simulink model "Copy_of_Carrier_Phase_Shift"  (R2021a)
settings: Solver=FixedStepAuto  StartTime=0.0  StopTime=0.01  FixedStep=1e-7  MaxStep=1e-7  RelTol=1e-6
InitFcn:
  | fsw=50e3;
  | ma=0.5;
  | ffund=100;
  | 
  | L1=63e-6;
  | L2=50e-6;
  | M=18e-6;
  | C1=12.2e-9;
  | C2=14.5e-9;
  | R=20;
  | 
  | sn3=C1*C2*M*R;
  | sd4=C1*C2*L1*L2+C1*C2*L1*M+C1*C2*L2*M;
  | sd3= C1*C2*L1*R+ C1*C2*M*R;
  | sd2= C1*L1+C2*L2+C1*M+C2*M;
  | sd1=C2*R;
  | sd0=1;
libraries: spsSeriesRLCBranchLib x9, spsDiodeLib x4, spsVoltageMeasurementLib x3, spsControlledVoltageSourceLib x1, spsCurrentMeasurementLib x1, dspsigops x1, spspowerguiLib x1
settings Model: Creator=enes_  LastModifiedBy=enes_
settings DataIOCC: SaveFormat=StructureWithTime  ReturnWorkspaceOutputs=off

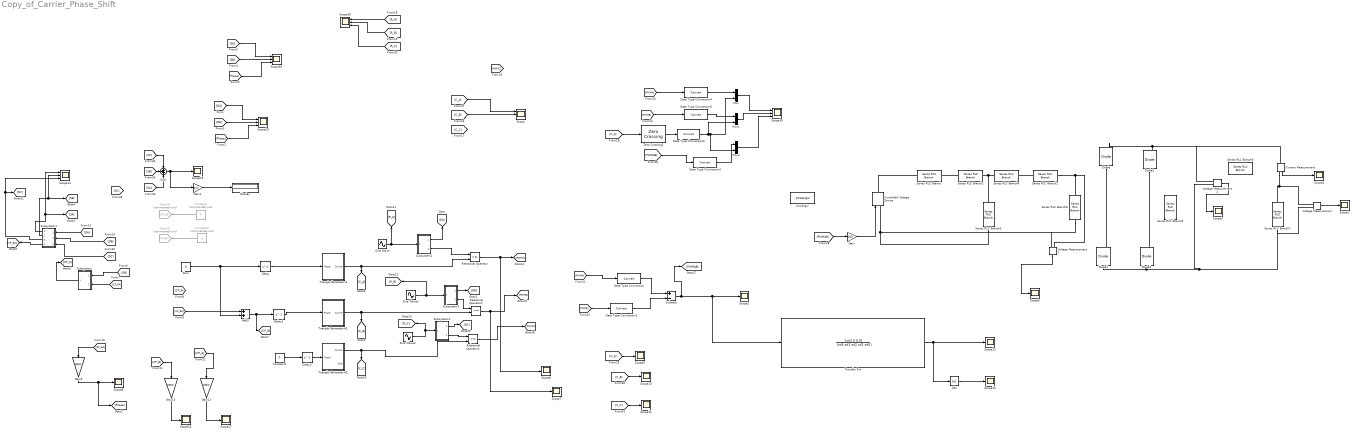
== system Copy_of_Carrier_Phase_Shift ==
  Abs : Abs
  Add3 : Sum
  Constant : Constant  Commented=on  Value=0
  Constant1 : Constant  Value=0
  Constant2 : Constant  Commented=on  Value=pi
  Controlled Voltage Source : spsControlledVoltageSourceLib/Controlled Voltage Source  Initialize=on  Source_Type=AC  Amplitude=0  Phase=0  Frequency=0  Measurements=None
  Current Measurement : spsCurrentMeasurementLib/Current Measurement  PhasorSimulation=off  OutputType=Complex  PSBequivalent=0
  Data Type Conversion{,1..2,4..6} (6 alike) : DataTypeConversion
  Delay : Delay  DelayLength=1
  Delay1 : Delay  DelayLength=1
  Delay2 : Delay  DelayLength=1
  Diode{,1..3} (4 alike) : spsDiodeLib/Diode  Ron=0.001  Lon=0  Vf=0.8  IC=0  UseSnubber=0  Rs=500  Cs=250e-9  Measurements=on
  Display : Display
  Gain : Gain  Gain=100
  Gain1 : Gain  Gain=pi/2
  Gain12 : Gain  Gain=180/pi
  Gain13 : Gain  Gain=180/pi
  Gain9 : Gain  Gain=180/pi
  Goto18 : Goto  Commented=on  GotoTag=CP_A
  Goto19 : Goto  Commented=on  GotoTag=CP_BA
  Mux : Mux  Inputs=2
  Mux1 : Mux  Inputs=2
  Mux2 : Mux  Inputs=2
  Relational Operator : RelationalOperator  OutDataTypeStr=boolean  RndMeth=Simplest
  Relational Operator1 : RelationalOperator  OutDataTypeStr=boolean  RndMeth=Simplest
  Relational Operator2 : RelationalOperator  OutDataTypeStr=boolean  RndMeth=Simplest
  Scope{,14,29..30,38..39} (6 alike) : Scope  NumInputPorts=3
  Scope{1..13,15..17} (16 alike) : Scope
  Series RLC Branch : spsSeriesRLCBranchLib/Series RLC Branch  LConnTagsString=__new0  RConnTagsString=__new0  BranchType=C  Resistance=1  Inductance=1e-3  SetiL0=off  InitialCurrent=0  Capacitance=12.2e-9  Setx0=off  InitialVoltage=0  Measurements=None
  Series RLC Branch1 : spsSeriesRLCBranchLib/Series RLC Branch  LConnTagsString=__new0  RConnTagsString=__new0  BranchType=C  Resistance=1  Inductance=1e-3  SetiL0=off  InitialCurrent=0  Capacitance=14.5e-9  Setx0=off  InitialVoltage=0  Measurements=None
  Series RLC Branch2 : spsSeriesRLCBranchLib/Series RLC Branch  LConnTagsString=__new0  RConnTagsString=__new0  BranchType=L  Resistance=1  Inductance=63e-6  SetiL0=off  InitialCurrent=0  Capacitance=1e-6  Setx0=off  InitialVoltage=0  Measurements=None
  Series RLC Branch3 : spsSeriesRLCBranchLib/Series RLC Branch  LConnTagsString=__new0  RConnTagsString=__new0  BranchType=L  Resistance=1  Inductance=18e-6  SetiL0=off  InitialCurrent=0  Capacitance=1e-6  Setx0=off  InitialVoltage=0  Measurements=None
  Series RLC Branch4 : spsSeriesRLCBranchLib/Series RLC Branch  LConnTagsString=__new0  RConnTagsString=__new0  BranchType=L  Resistance=1  Inductance=50e-6  SetiL0=off  InitialCurrent=0  Capacitance=1e-6  Setx0=off  InitialVoltage=0  Measurements=None
  Series RLC Branch5 : spsSeriesRLCBranchLib/Series RLC Branch  LConnTagsString=__new0  RConnTagsString=__new0  BranchType=C  Resistance=1  Inductance=1e-3  SetiL0=off  InitialCurrent=0  Capacitance=100e-6  Setx0=off  InitialVoltage=0  Measurements=None
  Series RLC Branch6 : spsSeriesRLCBranchLib/Series RLC Branch  LConnTagsString=__new0  RConnTagsString=__new0  BranchType=L  Resistance=1  Inductance=500e-6  SetiL0=off  InitialCurrent=0  Capacitance=14.5e-9  Setx0=off  InitialVoltage=0  Measurements=None
  Series RLC Branch7 : spsSeriesRLCBranchLib/Series RLC Branch  LConnTagsString=__new0  RConnTagsString=__new0  BranchType=R  Resistance=40  Inductance=5e-3  SetiL0=off  InitialCurrent=0  Capacitance=1e-6  Setx0=off  InitialVoltage=0  Measurements=None
  Series RLC Branch8 : spsSeriesRLCBranchLib/Series RLC Branch  LConnTagsString=__new0  RConnTagsString=__new0  BranchType=R  Resistance=40  Inductance=5e-3  SetiL0=off  InitialCurrent=0  Capacitance=1e-6  Setx0=off  InitialVoltage=0  Measurements=None
  Sine Wave : Sin  Amplitude=ma  Frequency=2*pi*ffund  SampleTime=0
  Sine Wave1 : Sin  Amplitude=ma  Frequency=2*pi*ffund  Phase=2*pi/3  SampleTime=0
  Sine Wave2 : Sin  Amplitude=ma  Frequency=2*pi*ffund  Phase=-2*pi/3  SampleTime=0
  Subsystem : Subsystem
  Subsystem1 : Subsystem
  Subsystem2 : Subsystem
  Subsystem3 : Subsystem
  Subsystem4 : Subsystem
  Subtract : Sum  Inputs=+-
  Sum : Sum  Inputs=+++
  Transfer Fcn : TransferFcn  Numerator=[sn3 0 0 0]  Denominator=[sd4 sd3 sd2 sd1 sd0]
  Triangle Generator-A : Subsystem
  Triangle Generator-A1 : Subsystem
  Triangle Generator-A2 : Subsystem
  Voltage Measurement : spsVoltageMeasurementLib/Voltage Measurement  PhasorSimulation=off  OutputType=Complex  PSBequivalent=0
  Voltage Measurement1 : spsVoltageMeasurementLib/Voltage Measurement  PhasorSimulation=off  OutputType=Complex  PSBequivalent=0
  Voltage Measurement2 : spsVoltageMeasurementLib/Voltage Measurement  PhasorSimulation=off  OutputType=Complex  PSBequivalent=0
  Zero : Constant  Value=0  OutDataTypeStr=Inherit: Inherit via back propagation
  Zero Crossing2 : dspsigops/Zero Crossing  InputProcessing=Columns as channels (frame based)
      settings: SourceProductBaseCode=DS
  powergui : spspowerguiLib/powergui  Priority=1  SimulationMode=Continuous  SampleTime=50e-6  frequency=60  Iterations=50  frequencyindice=0  Pbase=100e6  ErrMax=1e-4  UnitsV=kV  UnitsW=MW  buscounter=0  FunctionMessages=off  echomessages=off  EnableUseOfTLC=off  CurrentSourceSwitches=off  DisableSnubberDevices=off  DisableRonSwitches=off  DisableVfSwitches=off  DisplayEquations=off  AutomaticDiscreteSolvers=off  SolverType=Tustin/Backward Euler (TBE)  Interpol=off  ExternalGateDelay=off  methode=off  Ts=100  x0status=blocks  SPID=on  SwTol=0  HookPort=off  NonlinearTolerance=1e-4  nMaxIteration=100  ContinueOnMaxIteration=off  RestoreLinks=warning  ResistiveCurrentMeasurement=off  Frange=[0:2:500]  Ylog=off  Xlog=on  ShowGrid=off  save=off  variable=ZData  structure=0  ZoomFFT=off  StartTime=0.0  cycles=1  DisplayStyle=1  fundamental=60  FreqAxis=off  MaxFrequency=1000  frequencyindicesteady=1  RmsSteady=1  display=off
  wires:
  Triangle Generator-A2/1(Carrier) -> [C_C], Relational Operator2/2
  Relational Operator1/1 -> Scope7/1, [PWMB]
  Data Type Conversion/1 -> Subtract/1
  Data Type Conversion1/1 -> Subtract/2
  Constant1/1 -> Delay2/1
  Delay1/1 -> Triangle Generator-A1/1(Phase)
  Delay2/1 -> Triangle Generator-A2/1(Phase)
  Add3/1 -> [CP_B], Delay1/1
  Subtract/1 -> [PWMAB], Transfer Fcn/1, Scope2/1
  Delay/1 -> Triangle Generator-A/1(Phase)
  Gain9/1 -> [Phase], Scope8/1
  Gain12/1 -> Scope17/1
  Gain13/1 -> Scope16/1
  Sine Wave2/1 -> [R_C], Subsystem4/1(In1)
  [DA] -> Scope29/1
  [DB] -> Scope29/2
  [Phase] -> Scope29/3
  [SB] -> Scope30/2
  [Phase] -> Scope30/3
  [SA] -> Scope30/1
  Triangle Generator-A/1(Carrier) -> Relational Operator/2, [C_A]
  Zero Crossing2/1 -> Data Type Conversion6/1
  Subsystem/1(Out1) -> [CP_A]
  [SB] -> Subsystem/1(In1)
  [CP_BA] -> Subsystem/2(In2)
  [CP_BA] -> Add3/1
  [CP_BA] -> Gain9/1
  [CP_B] -> Gain13/1
  [CP_A] -> Gain12/1
  [DA] -> Subsystem1/1(In1)
  [DB] -> Subsystem1/2(In2)
  Subsystem1/1(Out1) -> Scope14/1, [SA]
  Subsystem1/4(Out3) -> [CP_BA]
  Subsystem2/1(Out1) -> [DA]
  Subsystem2/2(Out2) -> Relational Operator/1
  Triangle Generator-A1/1(Carrier) -> Relational Operator1/2, [C_B]
  Sine Wave1/1 -> [R_B], Subsystem3/1(In1)
  Subsystem3/1(Out1) -> [DB]
  Subsystem3/2(Out2) -> Relational Operator1/1
  Sine Wave/1 -> Subsystem2/1(In1), [R_A]
  [PWMA] -> Data Type Conversion4/1
  Mux/1 -> Scope39/1
  Mux1/1 -> Scope39/2
  Data Type Conversion4/1 -> Mux/1
  [PWMB] -> Data Type Conversion5/1
  Data Type Conversion5/1 -> Mux1/1
  Data Type Conversion6/1 -> Mux1/2, Mux2/2, Mux/2
  Relational Operator/1 -> Scope6/1, [PWMA]
  Relational Operator2/1 -> [PWMC]
  [PWMA] -> Data Type Conversion/1
  [PWMB] -> Data Type Conversion1/1
  [PWMAB] -> Data Type Conversion2/1
  Mux2/1 -> Scope39/3
  Data Type Conversion2/1 -> Mux2/1
  [C_A] -> Zero Crossing2/1
  [C_A] -> Scope/1
  [C_B] -> Scope/2
  [PWMAB] -> Gain/1
  Gain/1 -> Controlled Voltage Source/1
  Voltage Measurement/1 -> Scope1/1
  Voltage Measurement1/1 -> Scope3/1
  Current Measurement/1 -> Scope4/1
  Voltage Measurement2/1 -> Scope5/1
  [R_B] -> Scope38/2
  [R_C] -> Scope38/3
  [R_A] -> Scope38/1
  Constant/1 -> Goto18/1
  Constant2/1 -> Goto19/1
  [C_A] -> Scope9/1
  [C_B] -> Scope10/1
  [C_C] -> Scope11/1
  Transfer Fcn/1 -> Abs/1, Scope12/1
  Abs/1 -> Scope13/1
  Zero/1 -> Add3/2, Delay/1
  Subsystem1/2(Out2) -> Scope14/2, [SB]
  Subsystem4/2(Out2) -> Relational Operator2/1
  Subsystem4/1(Out1) -> [DC]
  [DC] -> Subsystem1/3(In3)
  Subsystem1/3(Out4) -> Scope14/3, [SC]
  [SA] -> Sum/3
  [SB] -> Sum/2
  [SC] -> Sum/1
  Sum/1 -> Gain1/1, Scope15/1
  Gain1/1 -> Display/1
  connections:
  Series RLC Branch/LConn1 -- Controlled Voltage Source/RConn1
  Series RLC Branch2/LConn1 -- Series RLC Branch/RConn1
  Series RLC Branch3/LConn1 -- Series RLC Branch4/LConn1 -- Series RLC Branch2/RConn1
  Series RLC Branch1/LConn1 -- Series RLC Branch4/RConn1
  Series RLC Branch1/RConn1 -- Series RLC Branch8/LConn1 -- Voltage Measurement2/LConn1
  Series RLC Branch3/RConn1 -- Series RLC Branch8/RConn1 -- Voltage Measurement2/LConn2 -- Controlled Voltage Source/LConn1
  Diode/RConn1 -- Current Measurement/LConn1 -- Voltage Measurement1/LConn1 -- Diode2/RConn1
  Diode1/LConn1 -- Voltage Measurement1/LConn2 -- Voltage Measurement/LConn2 -- Series RLC Branch7/RConn1 -- Diode3/LConn1
  Voltage Measurement/LConn1 -- Current Measurement/RConn1 -- Series RLC Branch7/LConn1
  Diode/LConn1 -- Diode1/RConn1
  Diode2/LConn1 -- Diode3/RConn1

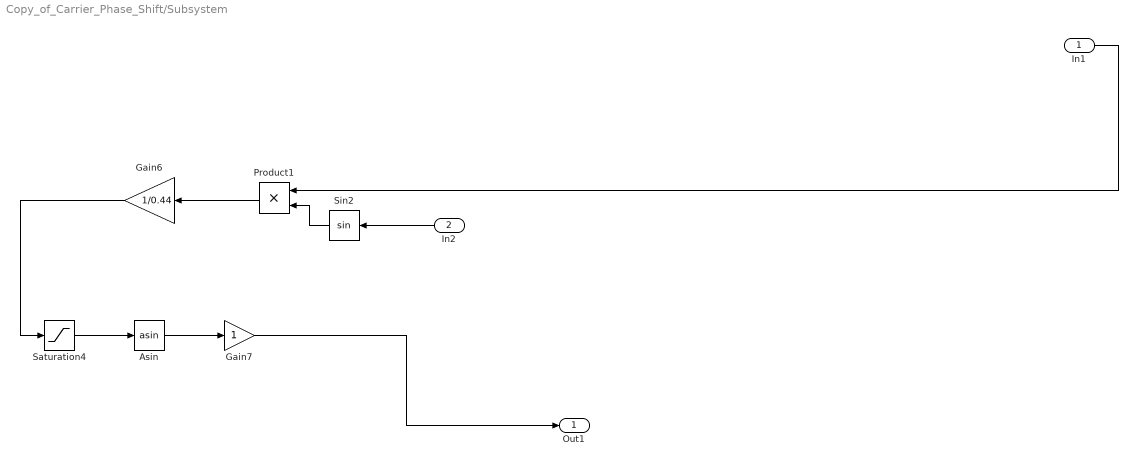
== system Copy_of_Carrier_Phase_Shift/Subsystem ==
  In1 : Inport
  In2 : Inport  Port=2
  Asin : Trigonometry  Operator=asin
  Gain6 : Gain  Gain=1/0.44
  Gain7 : Gain
  Product1 : Product
  Saturation4 : Saturate  UpperLimit=1  LowerLimit=-1
  Sin2 : Trigonometry
  Out1 : Outport
  wires:
  In2/1 -> Sin2/1
  Saturation4/1 -> Asin/1
  Gain7/1 -> Out1/1
  Gain6/1 -> Saturation4/1
  Asin/1 -> Gain7/1
  Product1/1 -> Gain6/1
  Sin2/1 -> Product1/2
  In1/1 -> Product1/1

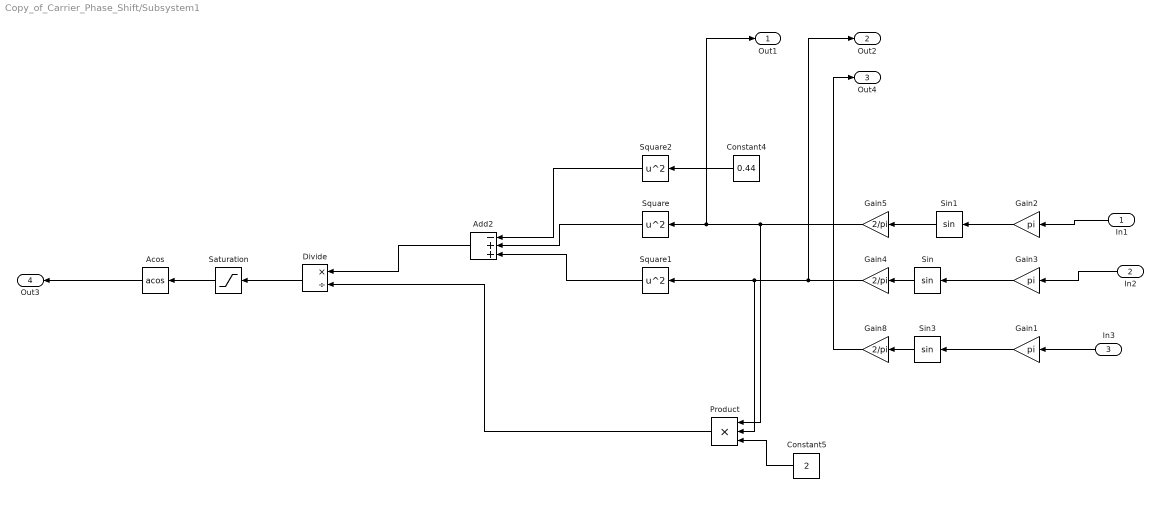
== system Copy_of_Carrier_Phase_Shift/Subsystem1 ==
  In1 : Inport
  In2 : Inport  Port=2
  In3 : Inport  Port=3
  Acos : Trigonometry  Operator=acos
  Add2 : Sum  Inputs=-++
  Constant4 : Constant  Value=0.44
  Constant5 : Constant  Value=2
  Divide : Product  Inputs=*/
  Gain1 : Gain  Gain=pi
  Gain2 : Gain  Gain=pi
  Gain3 : Gain  Gain=pi
  Gain4 : Gain  Gain=2/pi
  Gain5 : Gain  Gain=2/pi
  Gain8 : Gain  Gain=2/pi
  Product : Product  Inputs=3
  Saturation : Saturate  UpperLimit=1  LowerLimit=-1
  Sin : Trigonometry
  Sin1 : Trigonometry
  Sin3 : Trigonometry
  Square : Math  Operator=square  SaturateOnIntegerOverflow=on
  Square1 : Math  Operator=square  SaturateOnIntegerOverflow=on
  Square2 : Math  Operator=square  SaturateOnIntegerOverflow=on
  Out1 : Outport
  Out2 : Outport  Port=2
  Out4 : Outport  Port=3
  Out3 : Outport  Port=4
  wires:
  Gain4/1 -> Out2/1, Square1/1, Product/2
  Product/1 -> Divide/2
  Gain3/1 -> Sin/1
  Gain5/1 -> Out1/1, Square/1, Product/1
  Square/1 -> Add2/2
  Constant4/1 -> Square2/1
  Constant5/1 -> Product/3
  Square2/1 -> Add2/1
  Gain2/1 -> Sin1/1
  Square1/1 -> Add2/3
  Saturation/1 -> Acos/1
  Divide/1 -> Saturation/1
  Sin1/1 -> Gain5/1
  Add2/1 -> Divide/1
  Sin/1 -> Gain4/1
  In1/1 -> Gain2/1
  In2/1 -> Gain3/1
  Acos/1 -> Out3/1
  Sin3/1 -> Gain8/1
  Gain1/1 -> Sin3/1
  In3/1 -> Gain1/1
  Gain8/1 -> Out4/1

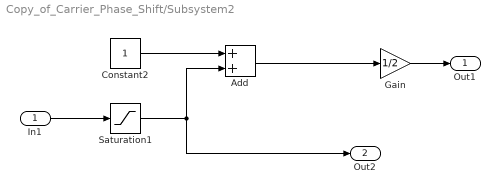
== system Copy_of_Carrier_Phase_Shift/Subsystem2 ==
  In1 : Inport
  Add : Sum
  Constant2 : Constant
  Gain : Gain  Gain=1/2
  Saturation1 : Saturate  UpperLimit=1  LowerLimit=-1
  Out1 : Outport
  Out2 : Outport  Port=2
  wires:
  Constant2/1 -> Add/1
  Add/1 -> Gain/1
  Gain/1 -> Out1/1
  In1/1 -> Saturation1/1
  Saturation1/1 -> Out2/1, Add/2

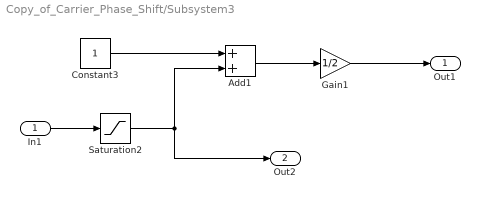
== system Copy_of_Carrier_Phase_Shift/Subsystem3 ==
  In1 : Inport
  Add1 : Sum
  Constant3 : Constant
  Gain1 : Gain  Gain=1/2
  Saturation2 : Saturate  UpperLimit=1  LowerLimit=-1
  Out1 : Outport
  Out2 : Outport  Port=2
  wires:
  Saturation2/1 -> Out2/1, Add1/2
  In1/1 -> Saturation2/1
  Constant3/1 -> Add1/1
  Add1/1 -> Gain1/1
  Gain1/1 -> Out1/1

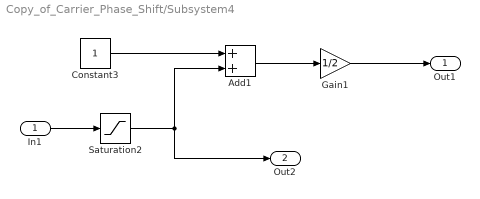
== system Copy_of_Carrier_Phase_Shift/Subsystem4 ==
  In1 : Inport
  Add1 : Sum
  Constant3 : Constant
  Gain1 : Gain  Gain=1/2
  Saturation2 : Saturate  UpperLimit=1  LowerLimit=-1
  Out1 : Outport
  Out2 : Outport  Port=2
  wires:
  Saturation2/1 -> Out2/1, Add1/2
  In1/1 -> Saturation2/1
  Constant3/1 -> Add1/1
  Add1/1 -> Gain1/1
  Gain1/1 -> Out1/1

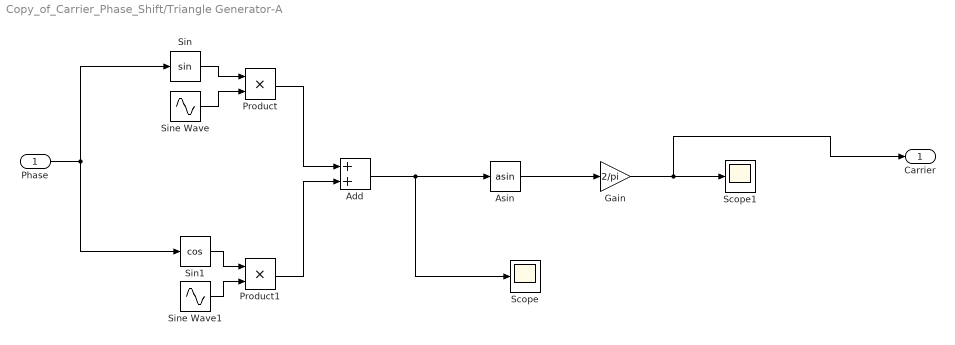
== system Copy_of_Carrier_Phase_Shift/Triangle Generator-A ==
  Phase : Inport
  Add : Sum
  Asin : Trigonometry  Operator=asin
  Gain : Gain  Gain=2/pi
  Product : Product
  Product1 : Product
  Scope : Scope
  Scope1 : Scope
  Sin : Trigonometry
  Sin1 : Trigonometry  Operator=cos
  Sine Wave : Sin  Frequency=2*pi*fsw  SampleTime=0
  Sine Wave1 : Sin  Frequency=2*pi*fsw  Phase=-pi/2  SampleTime=0
  Carrier : Outport
  wires:
  Sin/1 -> Product/1
  Sine Wave/1 -> Product/2
  Phase/1 -> Sin1/1, Sin/1
  Product/1 -> Add/1
  Asin/1 -> Gain/1
  Gain/1 -> Carrier/1, Scope1/1
  Sine Wave1/1 -> Product1/2
  Product1/1 -> Add/2
  Add/1 -> Asin/1, Scope/1
  Sin1/1 -> Product1/1

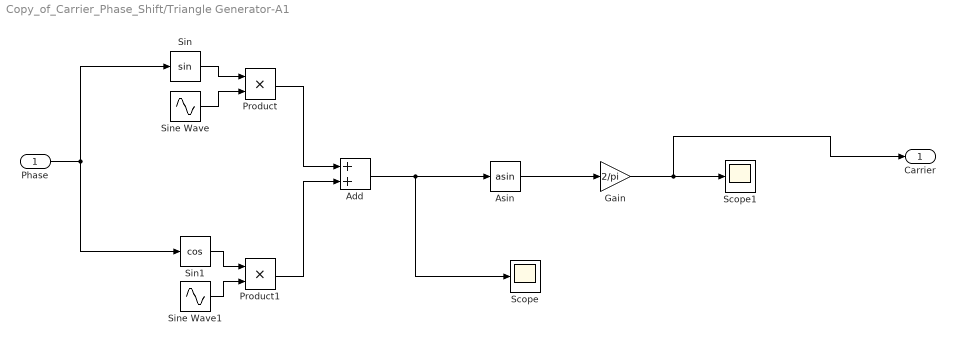
== system Copy_of_Carrier_Phase_Shift/Triangle Generator-A1 ==
  Phase : Inport
  Add : Sum
  Asin : Trigonometry  Operator=asin
  Gain : Gain  Gain=2/pi
  Product : Product
  Product1 : Product
  Scope : Scope
  Scope1 : Scope
  Sin : Trigonometry
  Sin1 : Trigonometry  Operator=cos
  Sine Wave : Sin  Frequency=2*pi*fsw  SampleTime=0
  Sine Wave1 : Sin  Frequency=2*pi*fsw  Phase=-pi/2  SampleTime=0
  Carrier : Outport
  wires:
  Sin/1 -> Product/1
  Sine Wave/1 -> Product/2
  Phase/1 -> Sin1/1, Sin/1
  Product/1 -> Add/1
  Asin/1 -> Gain/1
  Gain/1 -> Carrier/1, Scope1/1
  Sine Wave1/1 -> Product1/2
  Product1/1 -> Add/2
  Add/1 -> Asin/1, Scope/1
  Sin1/1 -> Product1/1

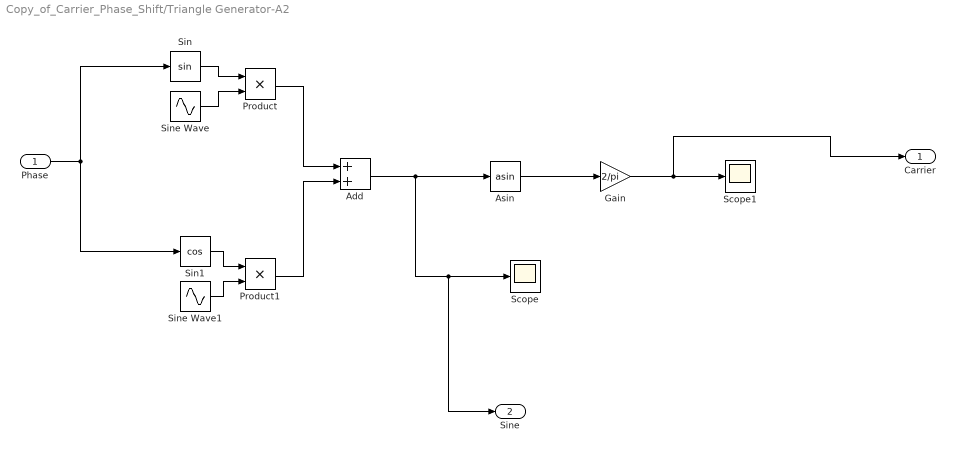
== system Copy_of_Carrier_Phase_Shift/Triangle Generator-A2 ==
  Phase : Inport
  Add : Sum
  Asin : Trigonometry  Operator=asin
  Gain : Gain  Gain=2/pi
  Product : Product
  Product1 : Product
  Scope : Scope
  Scope1 : Scope
  Sin : Trigonometry
  Sin1 : Trigonometry  Operator=cos
  Sine Wave : Sin  Frequency=2*pi*fsw  SampleTime=0
  Sine Wave1 : Sin  Frequency=2*pi*fsw  Phase=-pi/2  SampleTime=0
  Carrier : Outport
  Sine : Outport  Port=2
  wires:
  Sin/1 -> Product/1
  Sine Wave/1 -> Product/2
  Phase/1 -> Sin1/1, Sin/1
  Product/1 -> Add/1
  Asin/1 -> Gain/1
  Gain/1 -> Carrier/1, Scope1/1
  Sine Wave1/1 -> Product1/2
  Product1/1 -> Add/2
  Add/1 -> Asin/1, Sine/1, Scope/1
  Sin1/1 -> Product1/1
